simulink model "arduino_lab_R2017a"  (Simulink 8.9)
settings: Solver=VariableStepAuto  StartTime=0.0  StopTime=500  RelTol=1e-3  EnableMultiTasking=on
StartFcn:
  | clear all
libraries: realtime_pacer_lib x1
settings Model: Creator=johnh  LastModifiedBy=Sergio
settings DataIOCC: LimitDataPoints=off  SaveFormat=Dataset  SignalLoggingSaveFormat=Dataset
settings DebuggingCC: UnderspecifiedInitializationDetection=Simplified  MergeDetectMultiDrivingBlocksExec=error  FcnCallInpInsideContextMsg=error  StateNameClashWarn=none
settings HardwareCC: ProdBitPerPointer=64  ProdBitPerSizeT=64  ProdBitPerPtrDiffT=64  ProdLargestAtomicFloat=Float  ProdIntDivRoundTo=Zero  ProdEndianess=LittleEndian  ProdWordSize=64  ProdHWDeviceType=Intel->x86-64 (Windows64)
settings ModelReferenceCC: PropagateSignalLabelsOutOfModel=on
settings GRTTargetCC: CombineOutputUpdateFcns=on  GRTInterface=off

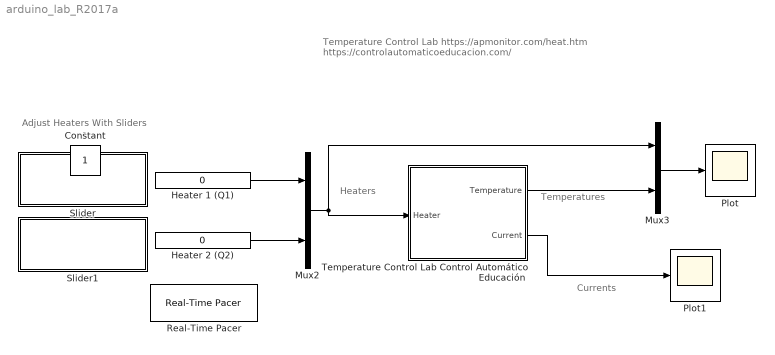
== system arduino_lab_R2017a ==
  note: Adjust Heaters With Sliders
  note: Temperature Control Lab
      | https://apmonitor.com/heat.htm
      | https://controlautomaticoeducacion.com/
  note: Heaters
  note: Temperatures
  note: Currents
  Heater 1 (Q1) : Constant  Value=0
  Heater 2 (Q2) : Constant  Value=0
  Mux2 : Mux  Inputs=2
  Mux3 : Mux  Inputs=2
  Plot : Scope
  Plot1 : Scope
  Real-Time Pacer : realtime_pacer_lib/Real-Time Pacer  simTimePerRealTime=1
  Slider : Subsystem  DialogController=hmiCreateDDGDialog  DialogControllerArgs=DataTag0  IsWebBlock=on  mask(MWDashboardBlock){webBlockId=6ba611ef-0cc5-4044-b83f-439e68c20d5f, webBlockType=slider, ShowInLibBrowser=on, ShowInitialText=on, HMISrcModelName=arduino_lab_R2017a}
      mask prompts: webBlockId "WebBlock Id"; webBlockType "WebBlock Type"; HMISrcModelName "Source Model"
      mask help: Set value to tune parameters or variables.
      mask Help: helpview([docroot '/mapfiles/simulink.map'], 'hmi_slider')
      mask Display:
      | if strcmp(get_param(bdroot(gcb),'BlockDiagramType'),'library')
      |  image([(matlabroot) '/toolbox/simulink/hmi/icons/Slider.png'])
      | end
  Slider1 : Subsystem  DialogController=hmiCreateDDGDialog  DialogControllerArgs=DataTag1  IsWebBlock=on  mask(MWDashboardBlock){webBlockId=ba1cd36f-4e7f-4531-b67e-e1a6f154e701, webBlockType=slider, ShowInLibBrowser=on, ShowInitialText=on, HMISrcModelName=arduino_lab_R2017a}
      mask prompts: webBlockId "WebBlock Id"; webBlockType "WebBlock Type"; HMISrcModelName "Source Model"
      mask help: Set value to tune parameters or variables.
      mask Help: helpview([docroot '/mapfiles/simulink.map'], 'hmi_slider')
      mask Display:
      | if strcmp(get_param(bdroot(gcb),'BlockDiagramType'),'library')
      |  image([(matlabroot) '/toolbox/simulink/hmi/icons/Slider.png'])
      | end
  Temperature Control Lab Control Automático Educación : Subsystem
      mask Display: image('tclab.jpg');
  1 : Constant  IOType=siggen
  Constant : Constant  IOType=siggen
  wires:
  Heater 1 (Q1)/1 -> Mux2/1
  Heater 2 (Q2)/1 -> Mux2/2
  Temperature Control Lab Control Automático Educación/1(Temperature) -> Mux3/2
  Mux3/1 -> Plot/1
  Mux2/1 -> Mux3/1, Temperature Control Lab Control Automático Educación/1(Heater)
  Temperature Control Lab Control Automático Educación/2(Current) -> Plot1/1

== system arduino_lab_R2017a/Slider ==

== system arduino_lab_R2017a/Slider1 ==

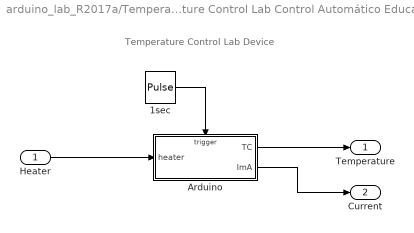
== system arduino_lab_R2017a/Temperature Control Lab Control Automático Educación ==
  note: Temperature Control Lab Device
  Heater : Inport
  1sec : DiscretePulseGenerator  PulseType=Time based  Period=1  PulseWidth=50
  Arduino : Subsystem  TreatAsAtomicUnit=on
  Temperature : Outport
  Current : Outport  Port=2
  wires:
  1sec/1 -> Arduino/Trigger
  Arduino/1(TC) -> Temperature/1
  Heater/1 -> Arduino/1(heater)
  Arduino/2(ImA) -> Current/1

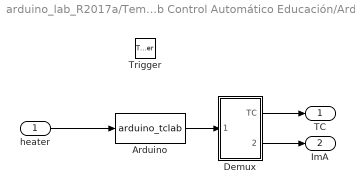
== system arduino_lab_R2017a/Temperature Control Lab Control Automático Educación/Arduino ==
  heater : Inport  LatchByDelayingOutsideSignal=on
  Trigger : TriggerPort  VariantControl=Variant
  Arduino : MATLABFcn  MATLABFcn=arduino_tclab
  Demux : Subsystem
  TC : Outport  InitialOutput=[25 25 25]
  ImA : Outport  Port=2  InitialOutput=[0 0]
  wires:
  heater/1 -> Arduino/1
  Arduino/1 -> Demux/1(In1)
  Demux/2(Out2) -> ImA/1
  Demux/1(TC) -> TC/1

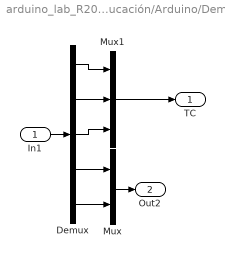
== system arduino_lab_R2017a/Temperature Control Lab Control Automático Educación/Arduino/Demux ==
  In1 : Inport
  Demux : Demux  Outputs=5
  Mux : Mux  Inputs=2
  Mux1 : Mux  Inputs=3
  TC : Outport
  Out2 : Outport  Port=2
  wires:
  Demux/5 -> Mux/2
  Demux/1 -> Mux1/1
  In1/1 -> Demux/1
  Demux/4 -> Mux/1
  Demux/2 -> Mux1/2
  Demux/3 -> Mux1/3
  Mux/1 -> Out2/1
  Mux1/1 -> TC/1
